simulink model "closed_loop_model_3_2"  (R2023b)
settings: Solver=ode1  StartTime=0.0  StopTime=30.0  FixedStep=0.001  RelTol=1e-3
values from neighbouring files (symbols this model uses):
  b = 0.02    [problem_3_2_inverted_pendulum.m]
  g = 9.81    [problem_3_2_inverted_pendulum.m]
  L = 0.15    [problem_3_2_inverted_pendulum.m]
  M = 0.05    [problem_3_2_inverted_pendulum.m]
  m = 0.04    [problem_3_2_inverted_pendulum.m]
settings Model: Creator=sarth  LastModifiedBy=sarth

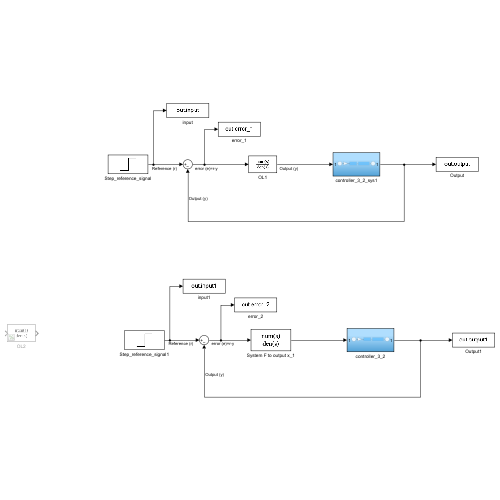
[thumbnail: Simulink's stored preview of the top-level diagram]
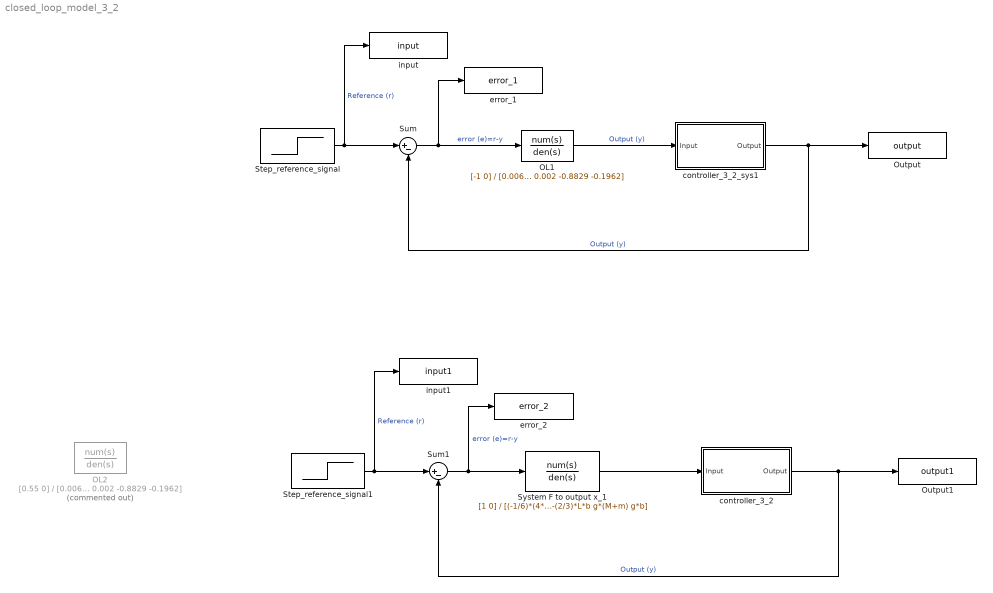
== system closed_loop_model_3_2 ==
  OL1 : TransferFcn  Numerator=[-1 0]  Denominator=[0.006 0.002 -0.8829 -0.1962]
  OL2 : TransferFcn  Commented=on  Numerator=[0.55 0]  Denominator=[0.006 0.002 -0.8829 -0.1962]
  Output : ToWorkspace  VariableName=output  SampleTime=-1
  Output1 : ToWorkspace  VariableName=output1  SampleTime=-1
  Step_reference_signal : Step  SampleTime=0
  Step_reference_signal1 : Step  SampleTime=0
  Sum : Sum  Inputs=|+-
  Sum1 : Sum  Inputs=|+-
  System F to output x_1 : TransferFcn  Numerator=[1 0]  Denominator=[(-1/6)*(4*M+m)*L -(2/3)*L*b g*(M+m) g*b]
  controller_3_2 : Subsystem
  controller_3_2_sys1 : Subsystem
  error_1 : ToWorkspace  VariableName=error_1  SampleTime=-1
  error_2 : ToWorkspace  VariableName=error_2  SampleTime=-1
  input : ToWorkspace  VariableName=input  SaveFormat=Timeseries  SampleTime=-1
  input1 : ToWorkspace  VariableName=input1  SampleTime=-1
  wires:
  Step_reference_signal/1 -> input/1, Sum/1  "Reference (r)"
  Sum/1 -> OL1/1, error_1/1  "error (e)=r-y"
  OL1/1 -> controller_3_2_sys1/1(Input)  "Output (y)"
  Sum1/1 -> System F to output x_1/1, error_2/1  "error (e)=r-y"
  controller_3_2/1(Output) -> Sum1/2, Output1/1  "Output (y)"
  Step_reference_signal1/1 -> input1/1, Sum1/1  "Reference (r)"
  System F to output x_1/1 -> controller_3_2/1(Input)
  controller_3_2_sys1/1(Output) -> Sum/2, Output/1  "Output (y)"

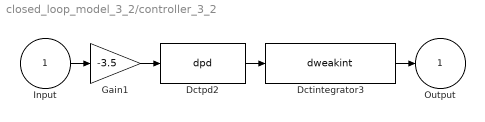
== system closed_loop_model_3_2/controller_3_2 ==
  Input : Inport
  Dctintegrator3 : S-Function  FunctionName=dweakint  Parameters=f_num, 0.001  SFunctionDeploymentMode=off  EnableBusSupport=off  mask(dctools){f_num=1}
      mask prompts: f_num "Zero [Hz]"
      mask help: This block implements a discrete time weak integrator filter.
      mask Display: disp('DCT integrator')
  Dctpd2 : S-Function  FunctionName=dpd  Parameters=kp, kv, 0.001  SFunctionDeploymentMode=off  EnableBusSupport=off  mask(dctools){kp=8, kv=0.09}
      mask help: This block implements a discrete time pd filter.
      mask Display: disp('DCT pd')
  Gain1 : Gain  Gain=-3.5
  Output : Outport
  wires:
  Input/1 -> Gain1/1
  Gain1/1 -> Dctpd2/1
  Dctpd2/1 -> Dctintegrator3/1
  Dctintegrator3/1 -> Output/1

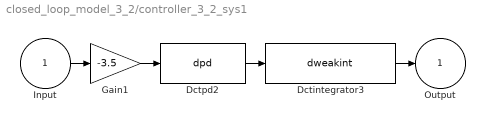
== system closed_loop_model_3_2/controller_3_2_sys1 ==
  Input : Inport
  Dctintegrator3 : S-Function  FunctionName=dweakint  Parameters=f_num, 0.001  SFunctionDeploymentMode=off  EnableBusSupport=off  mask(dctools){f_num=1}
      mask prompts: f_num "Zero [Hz]"
      mask help: This block implements a discrete time weak integrator filter.
      mask Display: disp('DCT integrator')
  Dctpd2 : S-Function  FunctionName=dpd  Parameters=kp, kv, 0.001  SFunctionDeploymentMode=off  EnableBusSupport=off  mask(dctools){kp=8, kv=0.09}
      mask help: This block implements a discrete time pd filter.
      mask Display: disp('DCT pd')
  Gain1 : Gain  Gain=-3.5
  Output : Outport
  wires:
  Input/1 -> Gain1/1
  Gain1/1 -> Dctpd2/1
  Dctpd2/1 -> Dctintegrator3/1
  Dctintegrator3/1 -> Output/1
